simulink model "lab1"  (R2017b)
settings: Solver=VariableStepAuto  StartTime=0.0  StopTime=100  RelTol=1e-3
settings Model: Creator=niquit  LastModifiedBy=niquit

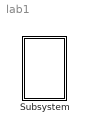
== system lab1 ==
  Subsystem : Subsystem  mask{Fi0=90, g=10, l=3, k=1, m=10}

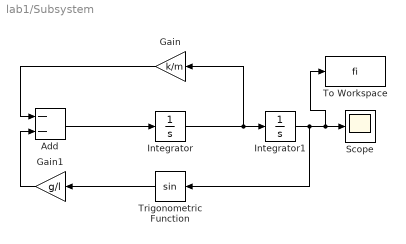
== system lab1/Subsystem ==
  Add : Sum  Inputs=--
  Gain : Gain  Gain=k/m
  Gain1 : Gain  Gain=g/l
  Integrator : Integrator
  Integrator1 : Integrator  InitialCondition=Fi0*pi/180
  Scope : Scope
  To Workspace : ToWorkspace  VariableName=fi  SampleTime=-1
  Trigonometric Function : Trigonometry
  wires:
  Trigonometric Function/1 -> Gain1/1
  Integrator1/1 -> Trigonometric Function/1, To Workspace/1, Scope/1
  Integrator/1 -> Gain/1, Integrator1/1
  Gain/1 -> Add/1
  Gain1/1 -> Add/2
  Add/1 -> Integrator/1
